simulink model "water_4hopper_VDF"  (Simulink 8.0)
settings: Solver=ode23  StartTime=0.0  StopTime=30  RelTol=1e-3
values from neighbouring files (symbols this model uses):
  alpha = 30    [SimParam_4VDF.m]
  Amp = leg_length    (= 0.0249)    [SimParam_4VDF.m]
  b_water = 0.5*C_d*S1*density    (= 0.405708731037)    [SimParam_4VDF.m]
  C_d = 0.703    [SimParam.m]    (also in SimParam_4VDF.m)
  density = 1000    [SimParam.m]    (also in SimParam_4VDF.m)
  frame_inertia = diag([Ix,Iy,Iz])    [SimParam.m]    (also in SimParam_4VDF.m)
  Fratio = 1/16    (= 0.0625)    [SimParam_4VDF.m]
  freq = 20    [SimParam.m]    (also in SimParam_4VDF.m = 60)
  g = 9.81    [SimParam.m]    (also in SimParam_4VDF.m)
  k_water = C_d*S1*density*g    (= 7.96000530294)    [SimParam_4VDF.m]
  leg_length = 0.06    [SimParam.m]    (also in SimParam_4VDF.m = 0.0249)
  Lx = frame_width/2*[-1 -1 1 1]'    [SimParam_4VDF.m]
  Lxmat = frame_width/2*[-1 0 0 0 ; 0 -1 0 0 ; 0 0 1 0 ; 0 0 0 1]    [SimParam_4VDF.m]
  Lz = frame_length/2*[-1 1 1 -1]'    [SimParam_4VDF.m]
  Lzmat = frame_length/2*[-1 0 0 0 ; 0 1 0 0 ; 0 0 1 0 ; 0 0 0 -1]    [SimParam_4VDF.m]
  mass = 0.1    [SimParam.m]    (also in SimParam_4VDF.m)
  mass_matrix = [mass 0 0; 0 Ix 0 ; 0 0 Iz]    [SimParam_4VDF.m]
  omega_0 = freq*ones(8,1)    [SimParam_4VDF.m]
  S1 = pi*r1^2    (= 0.00125663706144)    [SimParam.m]    (also in SimParam_4VDF.m = 0.00115422114093)
  S2 = pi*r2^2    (= 7.85398163397e-05)    [SimParam.m]    (also in SimParam_4VDF.m = 7.21388213081e-05)
  tau = 0.005    [SimParam_4VDF.m]
  wave = eps    [SimParam_4VDF.m]
  wavefreq = .5    (= 0.5)    [SimParam_4VDF.m]
undefined symbols (not defined in the file): amp, cw_FL_HL, cw_FR_FL, cw_FR_HR, cw_HR_HL, Filter_Coef, FL_HL_lag, FR_FL_lag, FR_HR_lag, HR_HL_lag, K_d, K_i, K_p, y_0
libraries: mblibv1 x34, dspstat3 x6, dspinverses x1
(part 1 of 2)
settings Model: Creator=Metti  LastModifiedBy=nitisht  SimulationMode=accelerator
settings SolverCC: ZeroCrossControl=DisableAll
settings DataIOCC: SignalLoggingSaveFormat=ModelDataLogs
settings DebuggingCC: FcnCallInpInsideContextMsg=EnableAllAsWarning
settings SimMechanicsCC: VisSampleTime=0.05  AutoFitVis=GROWTOFIT  LastVizWinPosition=[1 41 1600 759]  CamPosition=[-6.20117;3.01965;9.86212;]  CamTarget=[-0.265896;0.0450483;0.16365;]  CamUpVector=[0.0887544;0.966202;-0.242026;]  CamHeight=0.984746  VisBackgroundColor=[0.9;0.9;0.95;]  DefaultBodyColor=[1;0;0;]
settings ConfigurationSet: Description=SimMechanics 2G

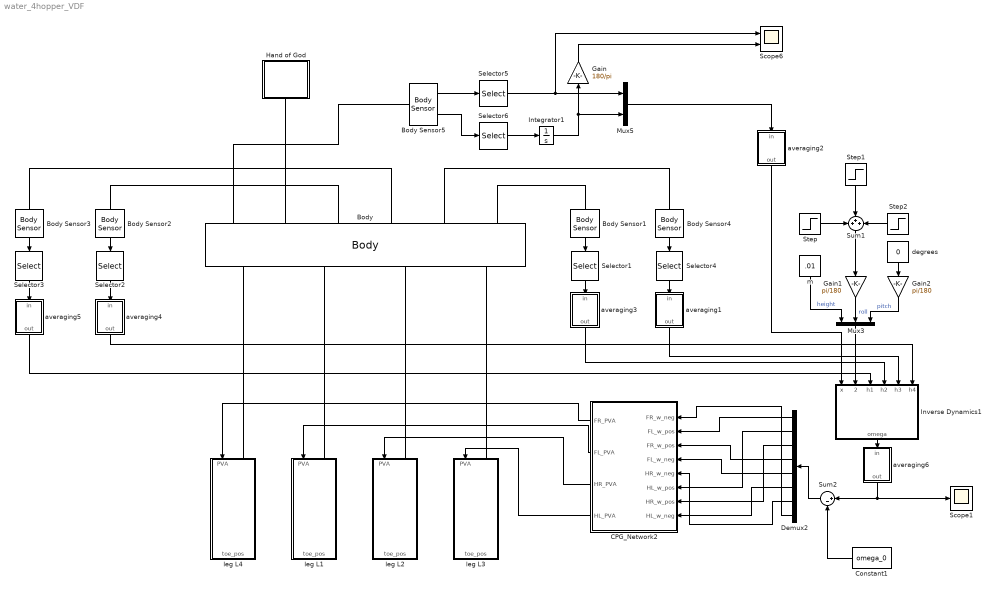
== system water_4hopper_VDF ==
  Body : mblibv1/Bodies/Body  LConnTagsString=CG|CS1|CS6|CS7|CS8|CS9  RConnTagsString=CS2|CS3|CS4|CS5  UpdateFromCAD=off  DialogClass=MechanicalBodyBlock  Mass=mass  MassUnits=kg  InertiaUnits=kg*m^2  Inertia=frame_inertia  Shape=Cylinder  ShapeDims=[1 1]  ShapeUnits=m  ShapeUse=false  Density=1  DensityUnits=kg/m^3  DensityUse=false  GraphicsMode=MACHINE_DEFAULT  BodyColorSelMode=MACHINE_DEFAULT  BodyColor=[1 0 0]  AttachedToCS=CG  CG=Left$CG$CG_pos$CS1$CS1$m$[0 0 0]$Euler X-Y-Z$deg$WORLD$true$none  WorkingFrames=Left$CS1$[0 0 0]$Adjoining$Adjoining$m$[0 0 0]$Euler X-Y-Z$deg$WORLD$true$none#Right$CS2$TR_FR$CS1$CS1$m$[0 0 0]$Euler X-Y-Z$deg$WORLD$true$none#Left$CS6$TR_FR$CS1$CS1$m$[0 0 0]$Euler X-Y-Z$deg$WORLD$true$none#Right$CS3$TR_FL$CS1$CS1$m$[0 0 0]$Euler X-Y-Z$deg$WORLD$true$none#Left$CS7$TR_FL$CS1$CS1$m$[0 0 0]$Euler X-Y-Z$deg$WORLD$true$none#Right$CS4$TR_HR$CS1$CS1$m$[0 0 0]$Euler X-Y-Z$deg$WORLD$true$none#Left$CS8$TR_HR$CS1$CS1$m$[0 0 0]$Euler X-Y-Z$deg$WORLD$true$none#Right$CS5$TR_HL$CS1$CS1$m$[0 0 0]$Euler X-Y-Z$deg$WORLD$true$none#Left$CS9$TR_HL$CS1$CS1$m$[0 0 0]$Euler X-Y-Z$deg$WORLD$true$none  CGPos=CG_pos  CGRot=[0 0 0]  CS0Pos=[]  CS0Rot=[]  CS1Pos=[0 0 0]  CS1Rot=[0 0 0]  CS2Pos=TR_FR  CS2Rot=[0 0 0]  CS3Pos=TR_FL  CS3Rot=[0 0 0]  CS4Pos=TR_HR  CS4Rot=[0 0 0]  CS5Pos=TR_HL  CS5Rot=[0 0 0]  CS6Pos=TR_FR  CS6Rot=[0 0 0]  CS7Pos=TR_FL  CS7Rot=[0 0 0]  CS8Pos=TR_HR  CS8Rot=[0 0 0]  CS9Pos=TR_HL  CS9Rot=[0 0 0]  CS10Pos=[]  CS10Rot=[]  CS11Pos=[]  CS11Rot=[]  CS12Pos=[]  CS12Rot=[]  CS13Pos=[]  CS13Rot=[]  CS14Pos=[]  CS14Rot=[]  CS15Pos=[]  CS15Rot=[]  CS16Pos=[]  CS16Rot=[]  CS17Pos=[]  CS17Rot=[]  CS18Pos=[]  CS18Rot=[]  CS19Pos=[]  CS19Rot=[]  CS20Pos=[]  CS20Rot=[]
  Body Sensor{1..4} (4 alike) : mblibv1/Sensors &  Actuators/Body Sensor  UpdateFromCAD=off  PhysicalDomain=Mechanical  PortType=blob  Muxed=on  Pose=off  Angle=on  AngleUnits=deg  ArcVelocity=off  ArcVelocityUnits=deg/s  ArcAcceleration=off  ArcAccelerationUnits=deg/s^2  CoordPosition=on  CoordPositionUnits=m  Velocity=off  VelocityUnits=m/s  Acceleration=off  AccelerationUnits=m/s^2  Quaternion=on  QuaternionDT=off  QuaternionDDT=off  QuaternionUnits=off  OutputVector=[1]  ActiveIO=on  Width=3  DialogClass=MechanicalSensorBlock  ReferenceFrame=Absolute (World)
  Body Sensor5 : mblibv1/Sensors &  Actuators/Body Sensor  UpdateFromCAD=off  PhysicalDomain=Mechanical  PortType=blob  Muxed=off  Pose=off  Angle=on  AngleUnits=deg  ArcVelocity=on  ArcVelocityUnits=rad/s  ArcAcceleration=off  ArcAccelerationUnits=deg/s^2  CoordPosition=on  CoordPositionUnits=m  Velocity=off  VelocityUnits=m/s  Acceleration=off  AccelerationUnits=m/s^2  Quaternion=on  QuaternionDT=off  QuaternionDDT=off  QuaternionUnits=off  OutputVector=[1]  ActiveIO=on  Width=6  DialogClass=MechanicalSensorBlock  ReferenceFrame=Absolute (World)
  CPG_Network2 : Subsystem
  Constant1 : Constant  Value=omega_0
  Demux2 : Demux  Outputs=8
  Gain : Gain  Gain=180/pi
  Gain1 : Gain  Gain=pi/180
  Gain2 : Gain  Gain=pi/180
  Hand of God : Subsystem
  Integrator1 : Integrator
  Inverse Dynamics1 : Subsystem
  Mux3 : Mux  Inputs=3
  Mux5 : Mux  Inputs=2
  Scope1 : Scope
      settings: TimeRange=30  YMin=5  YMax=105  SaveName=ball_position1
  Scope6 : Scope  NumInputPorts=2
      settings: TimeRange=30  YMin=-0.015~-17.5  YMax=0.065~15  SaveName=ball_position
  Selector{1..5} (5 alike) : Selector  InputPortWidth=3  IndexOptions=Index vector (dialog)  Indices=[2]  OutputSizes=1
  Selector6 : Selector  InputPortWidth=3  IndexOptions=Index vector (dialog)  Indices=[1 3]  OutputSizes=1
  Step : Step  Time=5  After=5  SampleTime=0
  Step1 : Step  Time=10  After=-10  SampleTime=0
  Step2 : Step  Time=15  After=5  SampleTime=0
  Sum1 : Sum  Inputs=+++
  Sum2 : Sum  Inputs=|+-
  averaging1 : Subsystem  mask{T_win=2*pi/freq*4, x_init=[y_0-leg_length, 0, 0]}
      mask prompts: T_win "window (s)"; x_init "Initial condition"
  averaging2 : Subsystem  mask{T_win=2*pi/freq*4, x_init=[y_0, 0, 0]}
      mask prompts: T_win "window (s)"; x_init "Initial condition"
  averaging3 : Subsystem  mask{T_win=2*pi/freq*4, x_init=[y_0-leg_length, 0, 0]}
      mask prompts: T_win "window (s)"; x_init "Initial condition"
  averaging4 : Subsystem  mask{T_win=2*pi/freq*4, x_init=[y_0-leg_length, 0, 0]}
      mask prompts: T_win "window (s)"; x_init "Initial condition"
  averaging5 : Subsystem  mask{T_win=2*pi/freq*4, x_init=[y_0-leg_length, 0, 0]}
      mask prompts: T_win "window (s)"; x_init "Initial condition"
  averaging6 : Subsystem  mask{T_win=2*pi/freq, x_init=omega_0}
      mask prompts: T_win "window (s)"; x_init "Initial condition"
  degrees : Constant  Value=0
  leg L1 : Subsystem  mask{seed=1}
      mask prompts: seed "random number seed"
  leg L2 : Subsystem  mask{seed=2}
      mask prompts: seed "random number seed"
  leg L3 : Subsystem  mask{seed=3}
      mask prompts: seed "random number seed"
  leg L4 : Subsystem  mask{seed=0}
      mask prompts: seed "random number seed"
  m : Constant  Value=.01
  wires:
  Body Sensor1/1 -> Selector1/1
  Body Sensor4/1 -> Selector4/1
  m/1 -> Mux3/1  "height"
  Mux3/1 -> Inverse Dynamics1/2(x_des)
  Selector5/1 -> Scope6/1, Mux5/1
  Integrator1/1 -> Mux5/2, Gain/1
  Body Sensor2/1 -> Selector2/1
  Body Sensor3/1 -> Selector3/1
  Body Sensor5/1 -> Selector5/1
  Body Sensor5/2 -> Selector6/1
  Selector6/1 -> Integrator1/1
  Constant1/1 -> Sum2/2
  Sum2/1 -> Demux2/1
  Demux2/1 -> CPG_Network2/2(FL_w_pos)
  Demux2/5 -> CPG_Network2/4(FL_w_neg)
  Demux2/2 -> CPG_Network2/6(HL_w_pos)
  Demux2/6 -> CPG_Network2/8(HL_w_neg)
  Demux2/3 -> CPG_Network2/7(HR_w_pos)
  Demux2/7 -> CPG_Network2/5(HR_w_neg)
  Demux2/4 -> CPG_Network2/3(FR_w_pos)
  Demux2/8 -> CPG_Network2/1(FR_w_neg)
  CPG_Network2/1(FR_PVA) -> leg L4/1(PVA)
  CPG_Network2/2(FL_PVA) -> leg L1/1(PVA)
  CPG_Network2/3(HR_PVA) -> leg L2/1(PVA)
  CPG_Network2/4(HL_PVA) -> leg L3/1(PVA)
  Gain/1 -> Scope6/2
  Gain1/1 -> Mux3/2  "roll"
  Gain2/1 -> Mux3/3  "pitch"
  Mux5/1 -> averaging2/1(in)
  averaging2/1(out) -> Inverse Dynamics1/1(x)
  Selector4/1 -> averaging1/1(in)
  Selector1/1 -> averaging3/1(in)
  Selector2/1 -> averaging4/1(in)
  Selector3/1 -> averaging5/1(in)
  averaging5/1(out) -> Inverse Dynamics1/3(h1)
  averaging4/1(out) -> Inverse Dynamics1/6(h4)
  averaging3/1(out) -> Inverse Dynamics1/4(h2)
  averaging1/1(out) -> Inverse Dynamics1/5(h3)
  Step/1 -> Sum1/1
  Step1/1 -> Sum1/2
  Step2/1 -> Sum1/3
  Inverse Dynamics1/1(omega) -> averaging6/1(in)
  averaging6/1(out) -> Sum2/1, Scope1/1
  degrees/1 -> Gain2/1
  Sum1/1 -> Gain1/1
  connections:
  Hand of God/RConn1 -- Body/LConn2
  Body/LConn6 -- Body Sensor1/LConn1
  Body/LConn5 -- Body Sensor4/LConn1
  Body/LConn1 -- Body Sensor5/LConn1
  leg L3/LConn1 -- Body/RConn4
  leg L2/LConn1 -- Body/RConn3
  leg L1/LConn1 -- Body/RConn2
  leg L4/LConn1 -- Body/RConn1
  Body/LConn3 -- Body Sensor2/LConn1
  Body/LConn4 -- Body Sensor3/LConn1

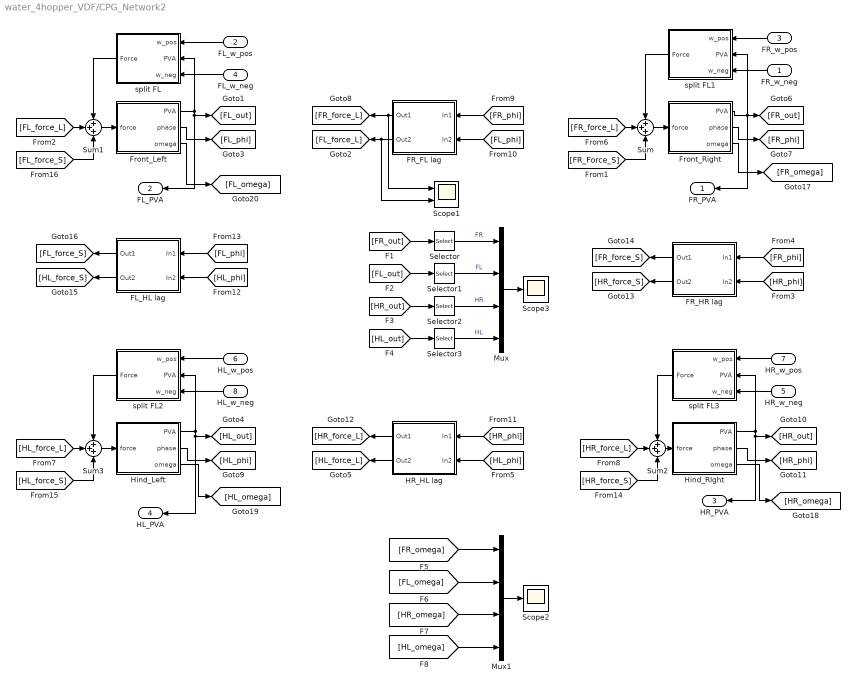
== system water_4hopper_VDF/CPG_Network2 ==
  FR_w_neg : Inport
  FL_w_pos : Inport  Port=2
  FR_w_pos : Inport  Port=3
  FL_w_neg : Inport  Port=4
  HR_w_neg : Inport  Port=5
  HL_w_pos : Inport  Port=6
  HR_w_pos : Inport  Port=7
  HL_w_neg : Inport  Port=8
  FL_HL lag : Subsystem  mask{d_phase=FL_HL_lag, coupling_weight=cw_FL_HL}
      mask prompts: d_phase "Phase Lag"; coupling_weight "Coupling Weight"
  FR_FL lag : Subsystem  mask{d_phase=FR_FL_lag, coupling_weight=cw_FR_FL}
      mask prompts: d_phase "Phase Lag"; coupling_weight "Coupling Weight"
  FR_HR lag : Subsystem  mask{d_phase=FR_HR_lag, coupling_weight=cw_FR_HR}
      mask prompts: d_phase "Phase Lag"; coupling_weight "Coupling Weight"
  Front_Left : Subsystem  mask{Amp=amp, Offset=0, init_phi=pi}
      mask prompts: Amp "Amplitude"; init_phi "Initial Phase"
  Front_Right : Subsystem  mask{Amp=amp, Offset=0, init_phi=0}
      mask prompts: Amp "Amplitude"; init_phi "Initial Phase"
  HR_HL lag : Subsystem  mask{d_phase=HR_HL_lag, coupling_weight=cw_HR_HL}
      mask prompts: d_phase "Phase Lag"; coupling_weight "Coupling Weight"
  Hind_Left : Subsystem  mask{Amp=amp, Offset=0, init_phi=0}
      mask prompts: Amp "Amplitude"; init_phi "Initial Phase"
  Hind_RIght : Subsystem  mask{Amp=amp, Offset=0, init_phi=pi}
      mask prompts: Amp "Amplitude"; init_phi "Initial Phase"
  Mux : Mux
  Mux1 : Mux
  Scope1 : Scope  NumInputPorts=2
      settings: ShowLegends=on  TimeRange=10  YMin=0~-5  YMax=2~5  SaveName=Output1
  Scope2 : Scope
      settings: ShowLegends=on  TimeRange=30  YMin=-20  YMax=130  SaveName=Output2
  Scope3 : Scope
      settings: ShowLegends=on  TimeRange=10  YMin=-0.025  YMax=0.025  SaveName=Output
  Selector{,1..3} (4 alike) : Selector  InputPortWidth=3  IndexOptions=Index vector (dialog)  Indices=[1]  OutputSizes=1
  Sum{,1..3} (4 alike) : Sum  Inputs=+++
  split FL : Subsystem
  split FL1 : Subsystem
  split FL2 : Subsystem
  split FL3 : Subsystem
  FR_PVA : Outport
  FL_PVA : Outport  Port=2
  HR_PVA : Outport  Port=3
  HL_PVA : Outport  Port=4
  wires:
  Mux/1 -> Scope3/1
  Front_Left/2(phase) -> [FL_phi]
  Front_Right/2(phase) -> [FR_phi]
  [FL_phi] -> FR_FL lag/2(In2)
  [FR_phi] -> FR_FL lag/1(In1)
  FR_FL lag/1(Out1) -> Scope1/1, [FR_force_L]
  FR_FL lag/2(Out2) -> Scope1/2, [FL_force_L]
  Front_Right/1(PVA) -> split FL1/2(PVA), FR_PVA/1, [FR_out]
  [FL_force_L] -> Sum1/2
  Sum1/1 -> Front_Left/1(force)
  Sum/1 -> Front_Right/1(force)
  [FR_force_L] -> Sum/2
  [FL_out] -> Selector1/1
  Selector1/1 -> Mux/2  "FL"
  Selector/1 -> Mux/1  "FR"
  [FR_out] -> Selector/1
  FR_w_pos/1 -> split FL1/1(w_pos)
  FR_w_neg/1 -> split FL1/3(w_neg)
  split FL1/1(Force) -> Sum/1
  FL_w_pos/1 -> split FL/1(w_pos)
  FL_w_neg/1 -> split FL/3(w_neg)
  Front_Left/1(PVA) -> FL_PVA/1, [FL_out], split FL/2(PVA)
  split FL/1(Force) -> Sum1/1
  Hind_Left/2(phase) -> [HL_phi]
  Hind_RIght/2(phase) -> [HR_phi]
  [HL_phi] -> HR_HL lag/2(In2)
  [HR_phi] -> HR_HL lag/1(In1)
  HR_HL lag/1(Out1) -> [HR_force_L]
  HR_HL lag/2(Out2) -> [HL_force_L]
  Hind_RIght/1(PVA) -> HR_PVA/1, [HR_out], split FL3/2(PVA)
  [HL_force_L] -> Sum3/2
  Sum3/1 -> Hind_Left/1(force)
  Sum2/1 -> Hind_RIght/1(force)
  [HR_force_L] -> Sum2/2
  HR_w_pos/1 -> split FL3/1(w_pos)
  HR_w_neg/1 -> split FL3/3(w_neg)
  split FL3/1(Force) -> Sum2/1
  HL_w_pos/1 -> split FL2/1(w_pos)
  HL_w_neg/1 -> split FL2/3(w_neg)
  Hind_Left/1(PVA) -> HL_PVA/1, [HL_out], split FL2/2(PVA)
  split FL2/1(Force) -> Sum3/1
  [HR_phi] -> FR_HR lag/2(In2)
  [FR_phi] -> FR_HR lag/1(In1)
  FR_HR lag/1(Out1) -> [FR_force_S]
  FR_HR lag/2(Out2) -> [HR_force_S]
  [HL_phi] -> FL_HL lag/2(In2)
  [FL_phi] -> FL_HL lag/1(In1)
  FL_HL lag/1(Out1) -> [FL_force_S]
  FL_HL lag/2(Out2) -> [HL_force_S]
  [HL_out] -> Selector3/1
  Selector3/1 -> Mux/4  "HL"
  Selector2/1 -> Mux/3  "HR"
  [HR_out] -> Selector2/1
  [FR_Force_S] -> Sum/3
  [HR_force_S] -> Sum2/3
  [HL_force_S] -> Sum3/3
  [FL_force_S] -> Sum1/3
  Front_Right/3(omega) -> [FR_omega]
  Hind_RIght/3(omega) -> [HR_omega]
  Hind_Left/3(omega) -> [HL_omega]
  Front_Left/3(omega) -> [FL_omega]
  Mux1/1 -> Scope2/1
  [FR_omega] -> Mux1/1
  [HL_omega] -> Mux1/4
  [HR_omega] -> Mux1/3
  [FL_omega] -> Mux1/2

== system water_4hopper_VDF/Hand of God ==
  Custom Joint : mblibv1/Joints/Custom Joint  LConnTagsString=__newl0|SA1  RConnTagsString=__newr0  UpdateFromCAD=off  NumSAPorts=1  CutJoint=off  MarkAsCut=off  Primitives=prismatic  PrimitiveProps=P1$World$[0 1 0]$Prismatic#R1$World$[1 0 0]$Revolute#R2$World$[0 0 1]$Revolute  DialogClass=JointBlock  R1Axis=[1 0 0]  R2Axis=[0 0 1]  R3Axis=[]  P1Axis=[0 1 0]  P2Axis=[]  P3Axis=[]  SAxis=[]
  Ground : mblibv1/Bodies/Ground  UpdateFromCAD=off  LeftPortType=env  RightPortType=workingframe  PhysicalDomain=Mechanical  DialogClass=GroundBlock  CoordPosition=[0 0 0]  CoordPositionUnits=m  StateVectorMgrId=3  MachineId=[4 0]  ShowEnvPort=on
  Joint Initial Condition : mblibv1/Sensors &  Actuators/Joint Initial Condition  UpdateFromCAD=off  LeftPortType=blob  RightPortType=blob  PhysicalDomain=mechanical  DialogClass=InitialConditionBlock  InitialConditions=P1$true$y_0$m$deg$0$m/s$deg/s#P2$false$0$m$deg$0$m/s$deg/s#P3$false$0$m$deg$0$m/s$deg/s#R1$true$0$m$deg$0$m/s$deg/s#R2$true$0$m$deg$0$m/s$deg/s#R3$false$10$m$deg$0$m/s$deg/s#S$false$0$m$deg$0$m/s$deg/s  P1PIC=y_0  P1VIC=0  P2PIC=0  P2VIC=0  P3PIC=0  P3VIC=0  R1PIC=0  R1VIC=0  R2PIC=0  R2VIC=0  R3PIC=0  R3VIC=0  SPIC=0  SVIC=0
  Joint Sensor : mblibv1/Sensors &  Actuators/Joint Sensor  UpdateFromCAD=off  PhysicalDomain=Mechanical  PortType=blob  Muxed=on  Pose=off  Angle=on  AngleUnits=deg  ArcVelocity=off  ArcVelocityUnits=deg/s  ArcAcceleration=off  ArcAccelerationUnits=deg/s^2  CoordPosition=on  CoordPositionUnits=m  Velocity=off  VelocityUnits=m/s  Acceleration=off  AccelerationUnits=m/s^2  Quaternion=on  QuaternionDT=off  QuaternionDDT=off  QuaternionUnits=off  OutputVector=[1]  ActiveIO=on  Width=1  DialogClass=MechanicalSensorBlock  Primitive=P1  Force=off  ForceUnits=N  Torque=off  TorqueUnits=N*m  ReferenceFrame=Absolute (World)  ReactionSensedSide=Base  ReactionReferenceFrame=Absolute (World)  ReactionForce=off  ReactionForceUnits=N  ReactionMoment=off  ReactionMomentUnits=N*m
  Joint Sensor1 : mblibv1/Sensors &  Actuators/Joint Sensor  UpdateFromCAD=off  PhysicalDomain=Mechanical  PortType=blob  Muxed=on  Pose=off  Angle=on  AngleUnits=deg  ArcVelocity=off  ArcVelocityUnits=deg/s  ArcAcceleration=off  ArcAccelerationUnits=deg/s^2  CoordPosition=off  CoordPositionUnits=m  Velocity=on  VelocityUnits=m/s  Acceleration=off  AccelerationUnits=m/s^2  Quaternion=on  QuaternionDT=off  QuaternionDDT=off  QuaternionUnits=off  OutputVector=[1]  ActiveIO=on  Width=1  DialogClass=MechanicalSensorBlock  Primitive=R1  Force=off  ForceUnits=N  Torque=off  TorqueUnits=N*m  ReferenceFrame=Absolute (World)  ReactionSensedSide=Base  ReactionReferenceFrame=Absolute (World)  ReactionForce=off  ReactionForceUnits=N  ReactionMoment=off  ReactionMomentUnits=N*m
  Joint Sensor2 : mblibv1/Sensors &  Actuators/Joint Sensor  UpdateFromCAD=off  PhysicalDomain=Mechanical  PortType=blob  Muxed=off  Pose=off  Angle=on  AngleUnits=deg  ArcVelocity=off  ArcVelocityUnits=deg/s  ArcAcceleration=off  ArcAccelerationUnits=deg/s^2  CoordPosition=on  CoordPositionUnits=m  Velocity=off  VelocityUnits=m/s  Acceleration=off  AccelerationUnits=m/s^2  Quaternion=on  QuaternionDT=off  QuaternionDDT=off  QuaternionUnits=off  OutputVector=[1]  ActiveIO=on  Width=1  DialogClass=MechanicalSensorBlock  Primitive=R2  Force=off  ForceUnits=N  Torque=off  TorqueUnits=N*m  ReferenceFrame=Absolute (World)  ReactionSensedSide=Base  ReactionReferenceFrame=Absolute (World)  ReactionForce=off  ReactionForceUnits=N  ReactionMoment=off  ReactionMomentUnits=N*m
  Machine Environment : mblibv1/Bodies/Machine Environment  PortType=env  PhysicalDomain=Mechanical  DialogTemplateClass=MECH.MachineEnvironment  SyncWhenCopied=off  Gravity=[0 -g 0]  GravityUnits=m/s^2  GravityAsSignal=off  Dimensionality=Auto-detect  AnalysisType=Forward dynamics  LinearAssemblyTolerance=1e-3  LinearAssemblyToleranceUnits=m  AngularAssemblyTolerance=1e-3  AngularAssemblyToleranceUnits=rad  ConstraintSolverType=Stabilizing  ConstraintRelTolerance=1e-4  ConstraintAbsTolerance=1e-4  UseRobustSingularityHandling=off  RedundancyAnalysisToleranceType=Automatically select tolerance  RedundancyAnalysisTolerance=1e-14  StatePerturbationType=Fixed  PerturbationSize=1e-5  VisualizeMachine=on  BodyVisualizationType=Use model default body geometries  BodyColorSelMode=Use model default  DefaultBodyColor=[1 0 0]
  Mechanical Branching Bar : mblibv1/Utilities/Mechanical Branching Bar  LConnTagsString=_newl0  RConnTagsString=__newr0|SA2|SA3|SA4  UpdateFromCAD=off  DialogClass=MechanicalBranchingBarBlock  NumSAPorts=4
  Scope : Scope  NumInputPorts=3
      settings: TimeRange=5  YMin=-0.01~-0.001~-6  YMax=0.02~0.0004~1  SaveName=mass_data
  Conn1 : PMIOPort  Port=1  Side=Right
  wires:
  Joint Sensor/1 -> Scope/1
  Joint Sensor1/1 -> Scope/2
  Joint Sensor2/1 -> Scope/3
  connections:
  Conn1/RConn1 -- Custom Joint/RConn1
  Joint Sensor1/LConn1 -- Mechanical Branching Bar/RConn3
  Ground/RConn1 -- Custom Joint/LConn1
  Machine Environment/RConn1 -- Ground/LConn1
  Joint Initial Condition/RConn1 -- Mechanical Branching Bar/RConn1
  Joint Sensor/LConn1 -- Mechanical Branching Bar/RConn2
  Custom Joint/LConn2 -- Mechanical Branching Bar/LConn1
  Joint Sensor2/LConn1 -- Mechanical Branching Bar/RConn4

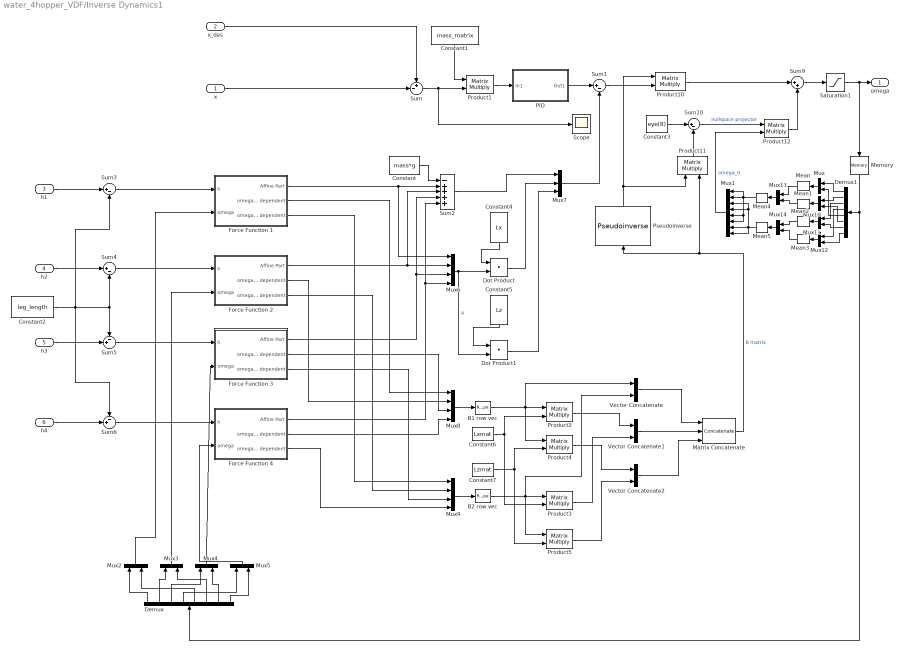
== system water_4hopper_VDF/Inverse Dynamics1 ==
  x : Inport
  x_des : Inport  Port=2
  h1 : Inport  Port=3
  h2 : Inport  Port=4
  h3 : Inport  Port=5
  h4 : Inport  Port=6
  B1 row vec : Reshape  OutputDimensionality=Row vector (2-D)  OutputDimensions=[1,2]
  B2 row vec : Reshape  OutputDimensionality=Row vector (2-D)  OutputDimensions=[1,2]
  Constant : Constant  Value=mass*g
  Constant1 : Constant  Value=mass_matrix
  Constant2 : Constant  Value=leg_length
  Constant3 : Constant  Value=eye(8)
  Constant4 : Constant  Value=Lx
  Constant5 : Constant  Value=Lz
  Constant6 : Constant  Value=Lxmat
  Constant7 : Constant  Value=Lzmat
  Demux : Demux  Outputs=8
  Demux1 : Demux  Outputs=8
  Dot Product : DotProduct  InputSameDT=on  OutDataTypeStr=Inherit: Inherit via internal rule
  Dot Product1 : DotProduct  InputSameDT=on  OutDataTypeStr=Inherit: Inherit via internal rule
  Force Function 1 : Subsystem
  Force Function 2 : Subsystem
  Force Function 3 : Subsystem
  Force Function 4 : Subsystem
  Matrix Concatenate : Concatenate  NumInputs=3  Mode=Multidimensional array
  Mean{,1..5} (6 alike) : dspstat3/Mean  run=off  reset_popup=None  InputProcessing=Columns as channels (frame based)  directionMode=Each column  dimension=1  treatSBRowAsCol=on  roiEnable=off  roiType=Rectangles  roiPortion=Entire ROI  roiOutput=Individual statistics for each ROI  roiFlag=off  outputDataTypeStr=Inherit: Same as accumulator  outputLastDataTypeStr=Inherit: Same as accumulator  outputMin=[]  outputMax=[]  roundingMode=Floor  overflowMode=off
  Memory : Memory  X0=omega_0
  Mux{,2..5,10..14} (10 alike) : Mux  Inputs=2
  Mux1 : Mux  Inputs=8
  Mux6 : Mux
  Mux7 : Mux  Inputs=3
  Mux8 : Mux
  Mux9 : Mux
  PID : Subsystem  mask{P=K_p, I=K_i, D=K_d, N=Filter_Coef}
      mask prompts: P "Proportional Gain"; I "Integral Gain"; D "Derivative Gain"; N "Filter Coefficient"
  Product{1..5,10..12} (8 alike) : Product  Multiplication=Matrix(*)  RndMeth=Zero
  Pseudoinverse : dspinverses/Pseudoinverse  wanterr=off
  Saturation1 : Saturate  UpperLimit=120  LowerLimit=10
  Scope : Scope
      settings: TimeRange=15  YMin=-0.01  YMax=0.09
  Sum : Sum  Inputs=+-|
  Sum{1,3..4,10} (4 alike) : Sum  Inputs=|+-
  Sum2 : Sum  Inputs=-++++
  Sum5 : Sum  Inputs=-+|
  Sum6 : Sum  Inputs=-+|
  Sum9 : Sum  Inputs=|++
  Vector Concatenate : Concatenate  ConcatenateDimension=2
  Vector Concatenate1 : Concatenate  ConcatenateDimension=2
  Vector Concatenate2 : Concatenate  ConcatenateDimension=2
  omega : Outport
  wires:
  Memory/1 -> Demux/1, Demux1/1
  PID/1(Out1) -> Sum1/1
  Sum/1 -> Scope/1, Product1/2
  x/1 -> Sum/2
  Pseudoinverse/1 -> Product11/1, Product10/1
  Sum1/1 -> Product10/2
  Product10/1 -> Sum9/1
  Product11/1 -> Sum10/2
  Constant3/1 -> Sum10/1
  Sum10/1 -> Product12/1  "nullspace projector"
  Product12/1 -> Sum9/2
  Mux1/1 -> Product12/2  "omega_0"
  Product1/1 -> PID/1(In1)
  Constant1/1 -> Product1/1
  Demux/1 -> Mux2/1
  Demux/5 -> Mux2/2
  Demux/2 -> Mux3/1
  Demux/6 -> Mux3/2
  Demux/3 -> Mux4/1
  Demux/7 -> Mux4/2
  Demux/4 -> Mux5/1
  Demux/8 -> Mux5/2
  Force Function 1/1(Affine Part) -> Mux6/1, Sum2/2
  Force Function 2/1(Affine Part) -> Sum2/3, Mux6/2
  Force Function 3/1(Affine Part) -> Mux6/3, Sum2/4
  Force Function 4/1(Affine Part) -> Mux6/4, Sum2/5
  Constant/1 -> Sum2/1
  Mux6/1 -> Dot Product/2, Dot Product1/2  "A"
  Constant4/1 -> Dot Product/1
  Constant5/1 -> Dot Product1/1
  Sum2/1 -> Mux7/1
  Dot Product/1 -> Mux7/2
  Dot Product1/1 -> Mux7/3
  Mux7/1 -> Sum1/2
  Force Function 1/2(omega1 dependent) -> Mux8/1
  Force Function 2/2(omega1 dependent) -> Mux8/2
  Force Function 3/2(omega1 dependent) -> Mux8/3
  Force Function 1/3(omega2 dependent) -> Mux9/1
  Force Function 2/3(omega2 dependent) -> Mux9/2
  Force Function 4/2(omega1 dependent) -> Mux8/4
  Force Function 3/3(omega2 dependent) -> Mux9/3
  Force Function 4/3(omega2 dependent) -> Mux9/4
  Mux8/1 -> B1 row vec/1
  Mux9/1 -> B2 row vec/1
  B1 row vec/1 -> Vector Concatenate/1, Product4/1, Product2/1
  B2 row vec/1 -> Vector Concatenate/2, Product5/1, Product3/1
  Constant6/1 -> Product3/2, Product2/2
  Constant7/1 -> Product4/2, Product5/2
  Product2/1 -> Vector Concatenate1/1
  Product3/1 -> Vector Concatenate1/2
  Product4/1 -> Vector Concatenate2/1
  Product5/1 -> Vector Concatenate2/2
  Vector Concatenate/1 -> Matrix Concatenate/1
  Vector Concatenate1/1 -> Matrix Concatenate/2
  Vector Concatenate2/1 -> Matrix Concatenate/3
  Matrix Concatenate/1 -> Product11/2, Pseudoinverse/1  "B matrix"
  Mux2/1 -> Force Function 1/2(omega)
  Mux3/1 -> Force Function 2/2(omega)
  Mux4/1 -> Force Function 3/2(omega)
  Mux5/1 -> Force Function 4/2(omega)
  h1/1 -> Sum3/1
  Sum3/1 -> Force Function 1/1(h)
  Sum4/1 -> Force Function 2/1(h)
  Sum5/1 -> Force Function 3/1(h)
  Sum6/1 -> Force Function 4/1(h)
  h2/1 -> Sum4/1
  h3/1 -> Sum5/2
  h4/1 -> Sum6/2
  Constant2/1 -> Sum3/2, Sum6/1, Sum5/1, Sum4/2
  x_des/1 -> Sum/1
  Sum9/1 -> Saturation1/1
  Saturation1/1 -> Memory/1, omega/1
  Demux1/1 -> Mux/1
  Mux/1 -> Mean/1
  Mux10/1 -> Mean1/1
  Mux11/1 -> Mean2/1
  Demux1/5 -> Mux/2
  Demux1/2 -> Mux10/1
  Demux1/6 -> Mux10/2
  Demux1/3 -> Mux11/1
  Demux1/7 -> Mux11/2
  Mux12/1 -> Mean3/1
  Demux1/4 -> Mux12/1
  Demux1/8 -> Mux12/2
  Mux13/1 -> Mean4/1
  Mean/1 -> Mux13/1
  Mean1/1 -> Mux13/2
  Mux14/1 -> Mean5/1
  Mean2/1 -> Mux14/1
  Mean3/1 -> Mux14/2
  Mean4/1 -> Mux1/6, Mux1/5, Mux1/2, Mux1/1
  Mean5/1 -> Mux1/8, Mux1/7, Mux1/4, Mux1/3

== system water_4hopper_VDF/averaging1 ==
  in : Inport
  Constant1 : Constant  Value=x_init
  Gain : Gain  Gain=1/T_win
  Integrator1 : Integrator
  Sum : Sum  Inputs=+-|
  Sum1 : Sum  Inputs=-+|
  Sum3 : Sum  Inputs=++|
  Transport Delay : TransportDelay  DelayTime=T_win
  out : Outport
  wires:
  in/1 -> Sum1/2
  Gain/1 -> Sum3/2
  Constant1/1 -> Sum3/1, Sum1/1
  Sum1/1 -> Integrator1/1
  Transport Delay/1 -> Sum/2
  Integrator1/1 -> Sum/1, Transport Delay/1
  Sum3/1 -> out/1
  Sum/1 -> Gain/1

== system water_4hopper_VDF/averaging2 ==
  in : Inport
  Constant1 : Constant  Value=x_init
  Gain : Gain  Gain=1/T_win
  Integrator1 : Integrator
  Sum : Sum  Inputs=+-|
  Sum1 : Sum  Inputs=-+|
  Sum3 : Sum  Inputs=++|
  Transport Delay : TransportDelay  DelayTime=T_win
  out : Outport
  wires:
  in/1 -> Sum1/2
  Gain/1 -> Sum3/2
  Constant1/1 -> Sum3/1, Sum1/1
  Sum1/1 -> Integrator1/1
  Transport Delay/1 -> Sum/2
  Integrator1/1 -> Sum/1, Transport Delay/1
  Sum3/1 -> out/1
  Sum/1 -> Gain/1

== system water_4hopper_VDF/averaging3 ==
  in : Inport
  Constant1 : Constant  Value=x_init
  Gain : Gain  Gain=1/T_win
  Integrator1 : Integrator
  Sum : Sum  Inputs=+-|
  Sum1 : Sum  Inputs=-+|
  Sum3 : Sum  Inputs=++|
  Transport Delay : TransportDelay  DelayTime=T_win
  out : Outport
  wires:
  in/1 -> Sum1/2
  Gain/1 -> Sum3/2
  Constant1/1 -> Sum3/1, Sum1/1
  Sum1/1 -> Integrator1/1
  Transport Delay/1 -> Sum/2
  Integrator1/1 -> Sum/1, Transport Delay/1
  Sum3/1 -> out/1
  Sum/1 -> Gain/1

== system water_4hopper_VDF/averaging4 ==
  in : Inport
  Constant1 : Constant  Value=x_init
  Gain : Gain  Gain=1/T_win
  Integrator1 : Integrator
  Sum : Sum  Inputs=+-|
  Sum1 : Sum  Inputs=-+|
  Sum3 : Sum  Inputs=++|
  Transport Delay : TransportDelay  DelayTime=T_win
  out : Outport
  wires:
  in/1 -> Sum1/2
  Gain/1 -> Sum3/2
  Constant1/1 -> Sum3/1, Sum1/1
  Sum1/1 -> Integrator1/1
  Transport Delay/1 -> Sum/2
  Integrator1/1 -> Sum/1, Transport Delay/1
  Sum3/1 -> out/1
  Sum/1 -> Gain/1

== system water_4hopper_VDF/averaging5 ==
  in : Inport
  Constant1 : Constant  Value=x_init
  Gain : Gain  Gain=1/T_win
  Integrator1 : Integrator
  Sum : Sum  Inputs=+-|
  Sum1 : Sum  Inputs=-+|
  Sum3 : Sum  Inputs=++|
  Transport Delay : TransportDelay  DelayTime=T_win
  out : Outport
  wires:
  in/1 -> Sum1/2
  Gain/1 -> Sum3/2
  Constant1/1 -> Sum3/1, Sum1/1
  Sum1/1 -> Integrator1/1
  Transport Delay/1 -> Sum/2
  Integrator1/1 -> Sum/1, Transport Delay/1
  Sum3/1 -> out/1
  Sum/1 -> Gain/1

== system water_4hopper_VDF/averaging6 ==
  in : Inport
  Constant1 : Constant  Value=x_init
  Gain : Gain  Gain=1/T_win
  Integrator1 : Integrator
  Sum : Sum  Inputs=+-|
  Sum1 : Sum  Inputs=-+|
  Sum3 : Sum  Inputs=++|
  Transport Delay : TransportDelay  DelayTime=T_win
  out : Outport
  wires:
  in/1 -> Sum1/2
  Gain/1 -> Sum3/2
  Constant1/1 -> Sum3/1, Sum1/1
  Sum1/1 -> Integrator1/1
  Transport Delay/1 -> Sum/2
  Integrator1/1 -> Sum/1, Transport Delay/1
  Sum3/1 -> out/1
  Sum/1 -> Gain/1

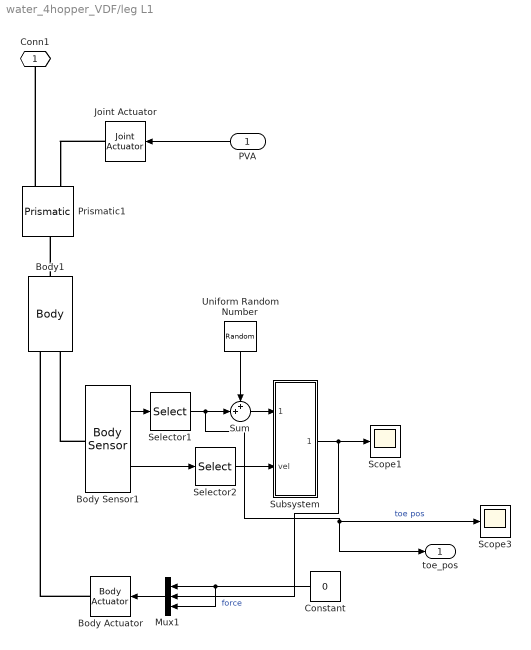
== system water_4hopper_VDF/leg L1 ==
  PVA : Inport
  Body Actuator : mblibv1/Sensors &  Actuators/Body Actuator  UpdateFromCAD=off  PhysicalDomain=Mechanical  PortType=blob  ActuationStyle=Force  AngleUnits=deg  ArcVelocityUnits=deg/s  ArcAccelerationUnits=deg/s^2  CoordPositionUnits=m  VelocityUnits=m/s  AccelerationUnits=m/s^2  ForceUnits=N  TorqueUnits=N*m  ActiveIO=on  Width=3  DialogClass=MechanicalActuatorBlock  ReferenceFrame=Absolute (World)  Angle=off  CoordPosition=on  Force=on  Torque=off
  Body Sensor1 : mblibv1/Sensors &  Actuators/Body Sensor  UpdateFromCAD=off  PhysicalDomain=Mechanical  PortType=blob  Muxed=off  Pose=off  Angle=on  AngleUnits=deg  ArcVelocity=off  ArcVelocityUnits=deg/s  ArcAcceleration=off  ArcAccelerationUnits=deg/s^2  CoordPosition=on  CoordPositionUnits=m  Velocity=on  VelocityUnits=m/s  Acceleration=off  AccelerationUnits=m/s^2  Quaternion=on  QuaternionDT=off  QuaternionDDT=off  QuaternionUnits=off  OutputVector=[1]  ActiveIO=on  Width=6  DialogClass=MechanicalSensorBlock  ReferenceFrame=Absolute (World)
  Body1 : mblibv1/Bodies/Body  LConnTagsString=CS1  RConnTagsString=CS2|CS3  UpdateFromCAD=off  DialogClass=MechanicalBodyBlock  Mass=0  MassUnits=kg  InertiaUnits=kg*m^2  Inertia=zeros(3)  Shape=Cylinder  ShapeDims=[1 1]  ShapeUnits=m  ShapeUse=false  Density=1  DensityUnits=kg/m^3  DensityUse=false  GraphicsMode=MACHINE_DEFAULT  BodyColorSelMode=MACHINE_DEFAULT  BodyColor=[1 0 0]  AttachedToCS=CG  CG=Left$CG$[0 -leg_length 0]$CS1$CS1$m$[0 0 0]$Euler X-Y-Z$deg$WORLD$false$none  WorkingFrames=Left$CS1$[0 0 0]$Adjoining$Adjoining$m$[0 0 0]$Euler X-Y-Z$deg$WORLD$true$none#Right$CS2$[0 -leg_length 0]$CS1$CS1$m$[0 0 0]$Euler X-Y-Z$deg$WORLD$true$none#Right$CS3$[0 -leg_length 0]$CS1$CS1$m$[0 0 0]$Euler X-Y-Z$deg$WORLD$true$none  CGPos=[0 -leg_length 0]  CGRot=[0 0 0]  CS0Pos=[]  CS0Rot=[]  CS1Pos=[0 0 0]  CS1Rot=[0 0 0]  CS2Pos=[0 -leg_length 0]  CS2Rot=[0 0 0]  CS3Pos=[0 -leg_length 0]  CS3Rot=[0 0 0]  CS4Pos=[]  CS4Rot=[]  CS5Pos=[]  CS5Rot=[]  CS6Pos=[]  CS6Rot=[]  CS7Pos=[]  CS7Rot=[]  CS8Pos=[]  CS8Rot=[]  CS9Pos=[]  CS9Rot=[]  CS10Pos=[]  CS10Rot=[]  CS11Pos=[]  CS11Rot=[]  CS12Pos=[]  CS12Rot=[]  CS13Pos=[]  CS13Rot=[]  CS14Pos=[]  CS14Rot=[]  CS15Pos=[]  CS15Rot=[]  CS16Pos=[]  CS16Rot=[]  CS17Pos=[]  CS17Rot=[]  CS18Pos=[]  CS18Rot=[]  CS19Pos=[]  CS19Rot=[]  CS20Pos=[]  CS20Rot=[]
  Constant : Constant  Value=0
  Joint Actuator : mblibv1/Sensors &  Actuators/Joint Actuator  UpdateFromCAD=off  PhysicalDomain=Mechanical  PortType=blob  ActuationStyle=Motion  AngleUnits=deg  ArcVelocityUnits=deg/s  ArcAccelerationUnits=deg/s^2  CoordPositionUnits=m  VelocityUnits=m/s  AccelerationUnits=m/s^2  ForceUnits=N  TorqueUnits=N*m  ActiveIO=on  Width=3  DialogClass=MechanicalActuatorBlock  Primitive=P1  ReferenceFrame=Absolute (World)
  Mux1 : Mux  Inputs=3
  Prismatic1 : mblibv1/Joints/Prismatic  LConnTagsString=__newl0|SA1  RConnTagsString=__newr0  UpdateFromCAD=off  NumSAPorts=1  CutJoint=off  MarkAsCut=off  Primitives=prismatic  PrimitiveProps=P1$World$[0 1 0]$prismatic  DialogClass=JointBlock  P1Axis=[0 1 0]
  Scope1 : Scope
      settings: SaveName=force_L
  Scope3 : Scope
      settings: SaveName=toe_position_L
  Selector1 : Selector  InputPortWidth=3  IndexOptions=Index vector (dialog)  Indices=[2]  OutputSizes=1
  Selector2 : Selector  InputPortWidth=3  IndexOptions=Index vector (dialog)  Indices=[2]  OutputSizes=1
  Subsystem : Subsystem
  Sum : Sum  Inputs=++|
  Uniform Random Number : UniformRandomNumber  Minimum=-wave  Maximum=wave  Seed=seed  SampleTime=1/wavefreq
  Conn1 : PMIOPort  Port=1  Side=Left
  toe_pos : Outport
  wires:
  Body Sensor1/2 -> Selector2/1
  Selector1/1 -> Sum/2, Scope3/1, toe_pos/1  "toe pos"
  Selector2/1 -> Subsystem/2(vel)
  Subsystem/1(force) -> Scope1/1, Mux1/2  "force"
  Mux1/1 -> Body Actuator/1
  Constant/1 -> Mux1/1, Mux1/3
  PVA/1 -> Joint Actuator/1
  Body Sensor1/1 -> Selector1/1
  Uniform Random Number/1 -> Sum/1
  Sum/1 -> Subsystem/1(pos)
  connections:
  Body1/LConn1 -- Prismatic1/RConn1
  Body Actuator/RConn1 -- Body1/RConn1
  Body Sensor1/LConn1 -- Body1/RConn2
  Prismatic1/LConn1 -- Conn1/RConn1
  Joint Actuator/RConn1 -- Prismatic1/LConn2

== system water_4hopper_VDF/leg L2 ==
  PVA : Inport
  Body Actuator : mblibv1/Sensors &  Actuators/Body Actuator  UpdateFromCAD=off  PhysicalDomain=Mechanical  PortType=blob  ActuationStyle=Force  AngleUnits=deg  ArcVelocityUnits=deg/s  ArcAccelerationUnits=deg/s^2  CoordPositionUnits=m  VelocityUnits=m/s  AccelerationUnits=m/s^2  ForceUnits=N  TorqueUnits=N*m  ActiveIO=on  Width=3  DialogClass=MechanicalActuatorBlock  ReferenceFrame=Absolute (World)  Angle=off  CoordPosition=on  Force=on  Torque=off
  Body Sensor1 : mblibv1/Sensors &  Actuators/Body Sensor  UpdateFromCAD=off  PhysicalDomain=Mechanical  PortType=blob  Muxed=off  Pose=off  Angle=on  AngleUnits=deg  ArcVelocity=off  ArcVelocityUnits=deg/s  ArcAcceleration=off  ArcAccelerationUnits=deg/s^2  CoordPosition=on  CoordPositionUnits=m  Velocity=on  VelocityUnits=m/s  Acceleration=off  AccelerationUnits=m/s^2  Quaternion=on  QuaternionDT=off  QuaternionDDT=off  QuaternionUnits=off  OutputVector=[1]  ActiveIO=on  Width=6  DialogClass=MechanicalSensorBlock  ReferenceFrame=Absolute (World)
  Body1 : mblibv1/Bodies/Body  LConnTagsString=CS1  RConnTagsString=CS2|CS3  UpdateFromCAD=off  DialogClass=MechanicalBodyBlock  Mass=0  MassUnits=kg  InertiaUnits=kg*m^2  Inertia=zeros(3)  Shape=Cylinder  ShapeDims=[1 1]  ShapeUnits=m  ShapeUse=false  Density=1  DensityUnits=kg/m^3  DensityUse=false  GraphicsMode=MACHINE_DEFAULT  BodyColorSelMode=MACHINE_DEFAULT  BodyColor=[1 0 0]  AttachedToCS=CG  CG=Left$CG$[0 -leg_length 0]$CS1$CS1$m$[0 0 0]$Euler X-Y-Z$deg$WORLD$false$none  WorkingFrames=Left$CS1$[0 0 0]$Adjoining$Adjoining$m$[0 0 0]$Euler X-Y-Z$deg$WORLD$true$none#Right$CS2$[0 -leg_length 0]$CS1$CS1$m$[0 0 0]$Euler X-Y-Z$deg$WORLD$true$none#Right$CS3$[0 -leg_length 0]$CS1$CS1$m$[0 0 0]$Euler X-Y-Z$deg$WORLD$true$none  CGPos=[0 -leg_length 0]  CGRot=[0 0 0]  CS0Pos=[]  CS0Rot=[]  CS1Pos=[0 0 0]  CS1Rot=[0 0 0]  CS2Pos=[0 -leg_length 0]  CS2Rot=[0 0 0]  CS3Pos=[0 -leg_length 0]  CS3Rot=[0 0 0]  CS4Pos=[]  CS4Rot=[]  CS5Pos=[]  CS5Rot=[]  CS6Pos=[]  CS6Rot=[]  CS7Pos=[]  CS7Rot=[]  CS8Pos=[]  CS8Rot=[]  CS9Pos=[]  CS9Rot=[]  CS10Pos=[]  CS10Rot=[]  CS11Pos=[]  CS11Rot=[]  CS12Pos=[]  CS12Rot=[]  CS13Pos=[]  CS13Rot=[]  CS14Pos=[]  CS14Rot=[]  CS15Pos=[]  CS15Rot=[]  CS16Pos=[]  CS16Rot=[]  CS17Pos=[]  CS17Rot=[]  CS18Pos=[]  CS18Rot=[]  CS19Pos=[]  CS19Rot=[]  CS20Pos=[]  CS20Rot=[]
  Constant : Constant  Value=0
  Joint Actuator : mblibv1/Sensors &  Actuators/Joint Actuator  UpdateFromCAD=off  PhysicalDomain=Mechanical  PortType=blob  ActuationStyle=Motion  AngleUnits=deg  ArcVelocityUnits=deg/s  ArcAccelerationUnits=deg/s^2  CoordPositionUnits=m  VelocityUnits=m/s  AccelerationUnits=m/s^2  ForceUnits=N  TorqueUnits=N*m  ActiveIO=on  Width=3  DialogClass=MechanicalActuatorBlock  Primitive=P1  ReferenceFrame=Absolute (World)
  Mux1 : Mux  Inputs=3
  Prismatic1 : mblibv1/Joints/Prismatic  LConnTagsString=__newl0|SA1  RConnTagsString=__newr0  UpdateFromCAD=off  NumSAPorts=1  CutJoint=off  MarkAsCut=off  Primitives=prismatic  PrimitiveProps=P1$World$[0 1 0]$prismatic  DialogClass=JointBlock  P1Axis=[0 1 0]
  Scope1 : Scope
      settings: SaveName=force_L
  Scope3 : Scope
      settings: SaveName=toe_position_L
  Selector1 : Selector  InputPortWidth=3  IndexOptions=Index vector (dialog)  Indices=[2]  OutputSizes=1
  Selector2 : Selector  InputPortWidth=3  IndexOptions=Index vector (dialog)  Indices=[2]  OutputSizes=1
  Subsystem : Subsystem
  Sum : Sum  Inputs=++|
  Uniform Random Number : UniformRandomNumber  Minimum=-wave  Maximum=wave  Seed=seed  SampleTime=1/wavefreq
  Conn1 : PMIOPort  Port=1  Side=Left
  toe_pos : Outport
  wires:
  Body Sensor1/2 -> Selector2/1
  Selector1/1 -> Sum/2, Scope3/1, toe_pos/1  "toe pos"
  Selector2/1 -> Subsystem/2(vel)
  Subsystem/1(force) -> Scope1/1, Mux1/2  "force"
  Mux1/1 -> Body Actuator/1
  Constant/1 -> Mux1/1, Mux1/3
  PVA/1 -> Joint Actuator/1
  Body Sensor1/1 -> Selector1/1
  Uniform Random Number/1 -> Sum/1
  Sum/1 -> Subsystem/1(pos)
  connections:
  Body1/LConn1 -- Prismatic1/RConn1
  Body Actuator/RConn1 -- Body1/RConn1
  Body Sensor1/LConn1 -- Body1/RConn2
  Prismatic1/LConn1 -- Conn1/RConn1
  Joint Actuator/RConn1 -- Prismatic1/LConn2

== system water_4hopper_VDF/leg L3 ==
  PVA : Inport
  Body Actuator : mblibv1/Sensors &  Actuators/Body Actuator  UpdateFromCAD=off  PhysicalDomain=Mechanical  PortType=blob  ActuationStyle=Force  AngleUnits=deg  ArcVelocityUnits=deg/s  ArcAccelerationUnits=deg/s^2  CoordPositionUnits=m  VelocityUnits=m/s  AccelerationUnits=m/s^2  ForceUnits=N  TorqueUnits=N*m  ActiveIO=on  Width=3  DialogClass=MechanicalActuatorBlock  ReferenceFrame=Absolute (World)  Angle=off  CoordPosition=on  Force=on  Torque=off
  Body Sensor1 : mblibv1/Sensors &  Actuators/Body Sensor  UpdateFromCAD=off  PhysicalDomain=Mechanical  PortType=blob  Muxed=off  Pose=off  Angle=on  AngleUnits=deg  ArcVelocity=off  ArcVelocityUnits=deg/s  ArcAcceleration=off  ArcAccelerationUnits=deg/s^2  CoordPosition=on  CoordPositionUnits=m  Velocity=on  VelocityUnits=m/s  Acceleration=off  AccelerationUnits=m/s^2  Quaternion=on  QuaternionDT=off  QuaternionDDT=off  QuaternionUnits=off  OutputVector=[1]  ActiveIO=on  Width=6  DialogClass=MechanicalSensorBlock  ReferenceFrame=Absolute (World)
  Body1 : mblibv1/Bodies/Body  LConnTagsString=CS1  RConnTagsString=CS2|CS3  UpdateFromCAD=off  DialogClass=MechanicalBodyBlock  Mass=0  MassUnits=kg  InertiaUnits=kg*m^2  Inertia=zeros(3)  Shape=Cylinder  ShapeDims=[1 1]  ShapeUnits=m  ShapeUse=false  Density=1  DensityUnits=kg/m^3  DensityUse=false  GraphicsMode=MACHINE_DEFAULT  BodyColorSelMode=MACHINE_DEFAULT  BodyColor=[1 0 0]  AttachedToCS=CG  CG=Left$CG$[0 -leg_length 0]$CS1$CS1$m$[0 0 0]$Euler X-Y-Z$deg$WORLD$false$none  WorkingFrames=Left$CS1$[0 0 0]$Adjoining$Adjoining$m$[0 0 0]$Euler X-Y-Z$deg$WORLD$true$none#Right$CS2$[0 -leg_length 0]$CS1$CS1$m$[0 0 0]$Euler X-Y-Z$deg$WORLD$true$none#Right$CS3$[0 -leg_length 0]$CS1$CS1$m$[0 0 0]$Euler X-Y-Z$deg$WORLD$true$none  CGPos=[0 -leg_length 0]  CGRot=[0 0 0]  CS0Pos=[]  CS0Rot=[]  CS1Pos=[0 0 0]  CS1Rot=[0 0 0]  CS2Pos=[0 -leg_length 0]  CS2Rot=[0 0 0]  CS3Pos=[0 -leg_length 0]  CS3Rot=[0 0 0]  CS4Pos=[]  CS4Rot=[]  CS5Pos=[]  CS5Rot=[]  CS6Pos=[]  CS6Rot=[]  CS7Pos=[]  CS7Rot=[]  CS8Pos=[]  CS8Rot=[]  CS9Pos=[]  CS9Rot=[]  CS10Pos=[]  CS10Rot=[]  CS11Pos=[]  CS11Rot=[]  CS12Pos=[]  CS12Rot=[]  CS13Pos=[]  CS13Rot=[]  CS14Pos=[]  CS14Rot=[]  CS15Pos=[]  CS15Rot=[]  CS16Pos=[]  CS16Rot=[]  CS17Pos=[]  CS17Rot=[]  CS18Pos=[]  CS18Rot=[]  CS19Pos=[]  CS19Rot=[]  CS20Pos=[]  CS20Rot=[]
  Constant : Constant  Value=0
  Joint Actuator : mblibv1/Sensors &  Actuators/Joint Actuator  UpdateFromCAD=off  PhysicalDomain=Mechanical  PortType=blob  ActuationStyle=Motion  AngleUnits=deg  ArcVelocityUnits=deg/s  ArcAccelerationUnits=deg/s^2  CoordPositionUnits=m  VelocityUnits=m/s  AccelerationUnits=m/s^2  ForceUnits=N  TorqueUnits=N*m  ActiveIO=on  Width=3  DialogClass=MechanicalActuatorBlock  Primitive=P1  ReferenceFrame=Absolute (World)
  Mux1 : Mux  Inputs=3
  Prismatic1 : mblibv1/Joints/Prismatic  LConnTagsString=__newl0|SA1  RConnTagsString=__newr0  UpdateFromCAD=off  NumSAPorts=1  CutJoint=off  MarkAsCut=off  Primitives=prismatic  PrimitiveProps=P1$World$[0 1 0]$prismatic  DialogClass=JointBlock  P1Axis=[0 1 0]
  Scope1 : Scope
      settings: SaveName=force_L
  Scope3 : Scope
      settings: SaveName=toe_position_L
  Selector1 : Selector  InputPortWidth=3  IndexOptions=Index vector (dialog)  Indices=[2]  OutputSizes=1
  Selector2 : Selector  InputPortWidth=3  IndexOptions=Index vector (dialog)  Indices=[2]  OutputSizes=1
  Subsystem : Subsystem
  Sum : Sum  Inputs=++|
  Uniform Random Number : UniformRandomNumber  Minimum=-wave  Maximum=wave  Seed=seed  SampleTime=1/wavefreq
  Conn1 : PMIOPort  Port=1  Side=Left
  toe_pos : Outport
  wires:
  Body Sensor1/2 -> Selector2/1
  Selector1/1 -> Sum/2, Scope3/1, toe_pos/1  "toe pos"
  Selector2/1 -> Subsystem/2(vel)
  Subsystem/1(force) -> Scope1/1, Mux1/2  "force"
  Mux1/1 -> Body Actuator/1
  Constant/1 -> Mux1/1, Mux1/3
  PVA/1 -> Joint Actuator/1
  Body Sensor1/1 -> Selector1/1
  Uniform Random Number/1 -> Sum/1
  Sum/1 -> Subsystem/1(pos)
  connections:
  Body1/LConn1 -- Prismatic1/RConn1
  Body Actuator/RConn1 -- Body1/RConn1
  Body Sensor1/LConn1 -- Body1/RConn2
  Prismatic1/LConn1 -- Conn1/RConn1
  Joint Actuator/RConn1 -- Prismatic1/LConn2

== system water_4hopper_VDF/leg L4 ==
  PVA : Inport
  Body Actuator : mblibv1/Sensors &  Actuators/Body Actuator  UpdateFromCAD=off  PhysicalDomain=Mechanical  PortType=blob  ActuationStyle=Force  AngleUnits=deg  ArcVelocityUnits=deg/s  ArcAccelerationUnits=deg/s^2  CoordPositionUnits=m  VelocityUnits=m/s  AccelerationUnits=m/s^2  ForceUnits=N  TorqueUnits=N*m  ActiveIO=on  Width=3  DialogClass=MechanicalActuatorBlock  ReferenceFrame=Absolute (World)  Angle=off  CoordPosition=on  Force=on  Torque=off
  Body Sensor1 : mblibv1/Sensors &  Actuators/Body Sensor  UpdateFromCAD=off  PhysicalDomain=Mechanical  PortType=blob  Muxed=off  Pose=off  Angle=on  AngleUnits=deg  ArcVelocity=off  ArcVelocityUnits=deg/s  ArcAcceleration=off  ArcAccelerationUnits=deg/s^2  CoordPosition=on  CoordPositionUnits=m  Velocity=on  VelocityUnits=m/s  Acceleration=off  AccelerationUnits=m/s^2  Quaternion=on  QuaternionDT=off  QuaternionDDT=off  QuaternionUnits=off  OutputVector=[1]  ActiveIO=on  Width=6  DialogClass=MechanicalSensorBlock  ReferenceFrame=Absolute (World)
  Body1 : mblibv1/Bodies/Body  LConnTagsString=CS1  RConnTagsString=CS2|CS3  UpdateFromCAD=off  DialogClass=MechanicalBodyBlock  Mass=0  MassUnits=kg  InertiaUnits=kg*m^2  Inertia=zeros(3)  Shape=Cylinder  ShapeDims=[1 1]  ShapeUnits=m  ShapeUse=false  Density=1  DensityUnits=kg/m^3  DensityUse=false  GraphicsMode=MACHINE_DEFAULT  BodyColorSelMode=MACHINE_DEFAULT  BodyColor=[1 0 0]  AttachedToCS=CG  CG=Left$CG$[0 -leg_length 0]$CS1$CS1$m$[0 0 0]$Euler X-Y-Z$deg$WORLD$false$none  WorkingFrames=Left$CS1$[0 0 0]$Adjoining$Adjoining$m$[0 0 0]$Euler X-Y-Z$deg$WORLD$true$none#Right$CS2$[0 -leg_length 0]$CS1$CS1$m$[0 0 0]$Euler X-Y-Z$deg$WORLD$true$none#Right$CS3$[0 -leg_length 0]$CS1$CS1$m$[0 0 0]$Euler X-Y-Z$deg$WORLD$true$none  CGPos=[0 -leg_length 0]  CGRot=[0 0 0]  CS0Pos=[]  CS0Rot=[]  CS1Pos=[0 0 0]  CS1Rot=[0 0 0]  CS2Pos=[0 -leg_length 0]  CS2Rot=[0 0 0]  CS3Pos=[0 -leg_length 0]  CS3Rot=[0 0 0]  CS4Pos=[]  CS4Rot=[]  CS5Pos=[]  CS5Rot=[]  CS6Pos=[]  CS6Rot=[]  CS7Pos=[]  CS7Rot=[]  CS8Pos=[]  CS8Rot=[]  CS9Pos=[]  CS9Rot=[]  CS10Pos=[]  CS10Rot=[]  CS11Pos=[]  CS11Rot=[]  CS12Pos=[]  CS12Rot=[]  CS13Pos=[]  CS13Rot=[]  CS14Pos=[]  CS14Rot=[]  CS15Pos=[]  CS15Rot=[]  CS16Pos=[]  CS16Rot=[]  CS17Pos=[]  CS17Rot=[]  CS18Pos=[]  CS18Rot=[]  CS19Pos=[]  CS19Rot=[]  CS20Pos=[]  CS20Rot=[]
  Constant : Constant  Value=0
  Joint Actuator : mblibv1/Sensors &  Actuators/Joint Actuator  UpdateFromCAD=off  PhysicalDomain=Mechanical  PortType=blob  ActuationStyle=Motion  AngleUnits=deg  ArcVelocityUnits=deg/s  ArcAccelerationUnits=deg/s^2  CoordPositionUnits=m  VelocityUnits=m/s  AccelerationUnits=m/s^2  ForceUnits=N  TorqueUnits=N*m  ActiveIO=on  Width=3  DialogClass=MechanicalActuatorBlock  Primitive=P1  ReferenceFrame=Absolute (World)
  Mux1 : Mux  Inputs=3
  Prismatic1 : mblibv1/Joints/Prismatic  LConnTagsString=__newl0|SA1  RConnTagsString=__newr0  UpdateFromCAD=off  NumSAPorts=1  CutJoint=off  MarkAsCut=off  Primitives=prismatic  PrimitiveProps=P1$World$[0 1 0]$prismatic  DialogClass=JointBlock  P1Axis=[0 1 0]
  Scope1 : Scope
      settings: SaveName=force_L
  Scope3 : Scope
      settings: SaveName=toe_position_L
  Selector1 : Selector  InputPortWidth=3  IndexOptions=Index vector (dialog)  Indices=[2]  OutputSizes=1
  Selector2 : Selector  InputPortWidth=3  IndexOptions=Index vector (dialog)  Indices=[2]  OutputSizes=1
  Subsystem : Subsystem
  Sum : Sum  Inputs=++|
  Uniform Random Number : UniformRandomNumber  Minimum=-wave  Maximum=wave  Seed=seed  SampleTime=1/wavefreq
  Conn1 : PMIOPort  Port=1  Side=Left
  toe_pos : Outport
  wires:
  Body Sensor1/2 -> Selector2/1
  Selector1/1 -> Sum/2, Scope3/1, toe_pos/1  "toe pos"
  Selector2/1 -> Subsystem/2(vel)
  Subsystem/1(force) -> Scope1/1, Mux1/2  "force"
  Mux1/1 -> Body Actuator/1
  Constant/1 -> Mux1/1, Mux1/3
  PVA/1 -> Joint Actuator/1
  Body Sensor1/1 -> Selector1/1
  Uniform Random Number/1 -> Sum/1
  Sum/1 -> Subsystem/1(pos)
  connections:
  Body1/LConn1 -- Prismatic1/RConn1
  Body Actuator/RConn1 -- Body1/RConn1
  Body Sensor1/LConn1 -- Body1/RConn2
  Prismatic1/LConn1 -- Conn1/RConn1
  Joint Actuator/RConn1 -- Prismatic1/LConn2

== system water_4hopper_VDF/CPG_Network2/FL_HL lag ==
  In1 : Inport
  In2 : Inport  Port=2
  Constant : Constant  Value=d_phase
  Gain : Gain  Gain=-1
  Sum : Sum  Inputs=--+
  sin : Fcn  Expr=coupling_weight*sin(u(1))
  Out1 : Outport
  Out2 : Outport  Port=2
  wires:
  Sum/1 -> sin/1
  sin/1 -> Gain/1, Out1/1
  Constant/1 -> Sum/2
  In1/1 -> Sum/1
  In2/1 -> Sum/3
  Gain/1 -> Out2/1

== system water_4hopper_VDF/CPG_Network2/FR_FL lag ==
  In1 : Inport
  In2 : Inport  Port=2
  Constant : Constant  Value=d_phase
  Gain : Gain  Gain=-1
  Sum : Sum  Inputs=--+
  sin : Fcn  Expr=coupling_weight*sin(u(1))
  Out1 : Outport
  Out2 : Outport  Port=2
  wires:
  Sum/1 -> sin/1
  sin/1 -> Gain/1, Out1/1
  Constant/1 -> Sum/2
  In1/1 -> Sum/1
  In2/1 -> Sum/3
  Gain/1 -> Out2/1

== system water_4hopper_VDF/CPG_Network2/FR_HR lag ==
  In1 : Inport
  In2 : Inport  Port=2
  Constant : Constant  Value=d_phase
  Gain : Gain  Gain=-1
  Sum : Sum  Inputs=--+
  sin : Fcn  Expr=coupling_weight*sin(u(1))
  Out1 : Outport
  Out2 : Outport  Port=2
  wires:
  Gain/1 -> Out2/1
  In2/1 -> Sum/3
  In1/1 -> Sum/1
  Constant/1 -> Sum/2
  sin/1 -> Out1/1, Gain/1
  Sum/1 -> sin/1

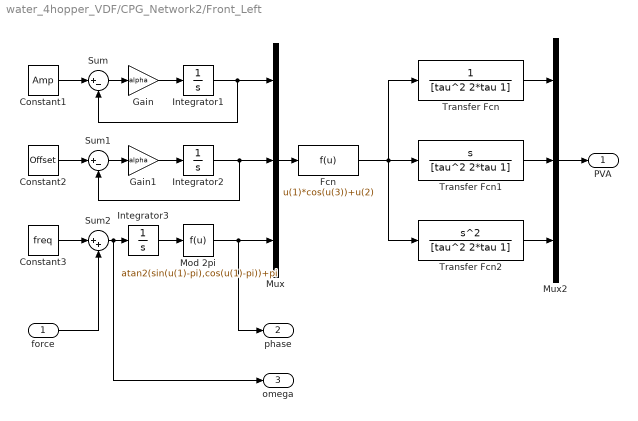
== system water_4hopper_VDF/CPG_Network2/Front_Left ==
  force : Inport
  Constant1 : Constant  Value=Amp
  Constant2 : Constant  Value=Offset
  Constant3 : Constant  Value=freq
  Fcn : Fcn  Expr=u(1)*cos(u(3))+u(2)
  Gain : Gain  Gain=alpha
  Gain1 : Gain  Gain=alpha
  Integrator1 : Integrator
  Integrator2 : Integrator
  Integrator3 : Integrator  InitialCondition=init_phi + 0.01*rand
  Mod 2pi : Fcn  Expr=atan2(sin(u(1)-pi),cos(u(1)-pi))+pi
  Mux : Mux  Inputs=3
  Mux2 : Mux  Inputs=3
  Sum : Sum  Inputs=|+-
  Sum1 : Sum  Inputs=|+-
  Sum2 : Sum  Inputs=|++
  Transfer Fcn : TransferFcn  Denominator=[tau^2 2*tau 1]
  Transfer Fcn1 : TransferFcn  Numerator=[1 0]  Denominator=[tau^2 2*tau 1]
  Transfer Fcn2 : TransferFcn  Numerator=[1 0 0]  Denominator=[tau^2 2*tau 1]
  PVA : Outport
  phase : Outport  Port=2
  omega : Outport  Port=3
  wires:
  Sum/1 -> Gain/1
  Integrator1/1 -> Sum/2, Mux/1
  Constant1/1 -> Sum/1
  Gain/1 -> Integrator1/1
  Sum1/1 -> Gain1/1
  Integrator2/1 -> Sum1/2, Mux/2
  Constant2/1 -> Sum1/1
  Gain1/1 -> Integrator2/1
  Mux/1 -> Fcn/1
  Mod 2pi/1 -> phase/1, Mux/3
  Integrator3/1 -> Mod 2pi/1
  Constant3/1 -> Sum2/1
  Sum2/1 -> omega/1, Integrator3/1
  force/1 -> Sum2/2
  Transfer Fcn2/1 -> Mux2/3
  Transfer Fcn/1 -> Mux2/1
  Transfer Fcn1/1 -> Mux2/2
  Fcn/1 -> Transfer Fcn2/1, Transfer Fcn/1, Transfer Fcn1/1
  Mux2/1 -> PVA/1

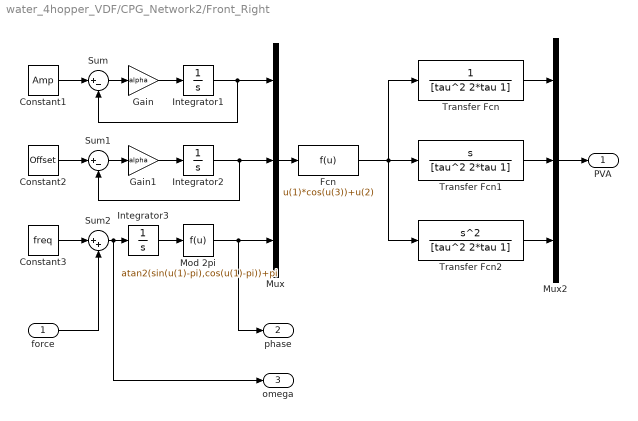
== system water_4hopper_VDF/CPG_Network2/Front_Right ==
  force : Inport
  Constant1 : Constant  Value=Amp
  Constant2 : Constant  Value=Offset
  Constant3 : Constant  Value=freq
  Fcn : Fcn  Expr=u(1)*cos(u(3))+u(2)
  Gain : Gain  Gain=alpha
  Gain1 : Gain  Gain=alpha
  Integrator1 : Integrator
  Integrator2 : Integrator
  Integrator3 : Integrator  InitialCondition=init_phi + 0.01*rand
  Mod 2pi : Fcn  Expr=atan2(sin(u(1)-pi),cos(u(1)-pi))+pi
  Mux : Mux  Inputs=3
  Mux2 : Mux  Inputs=3
  Sum : Sum  Inputs=|+-
  Sum1 : Sum  Inputs=|+-
  Sum2 : Sum  Inputs=|++
  Transfer Fcn : TransferFcn  Denominator=[tau^2 2*tau 1]
  Transfer Fcn1 : TransferFcn  Numerator=[1 0]  Denominator=[tau^2 2*tau 1]
  Transfer Fcn2 : TransferFcn  Numerator=[1 0 0]  Denominator=[tau^2 2*tau 1]
  PVA : Outport
  phase : Outport  Port=2
  omega : Outport  Port=3
  wires:
  Sum/1 -> Gain/1
  Integrator1/1 -> Sum/2, Mux/1
  Constant1/1 -> Sum/1
  Gain/1 -> Integrator1/1
  Sum1/1 -> Gain1/1
  Integrator2/1 -> Sum1/2, Mux/2
  Constant2/1 -> Sum1/1
  Gain1/1 -> Integrator2/1
  Mux/1 -> Fcn/1
  Mod 2pi/1 -> phase/1, Mux/3
  Integrator3/1 -> Mod 2pi/1
  Constant3/1 -> Sum2/1
  Sum2/1 -> omega/1, Integrator3/1
  force/1 -> Sum2/2
  Transfer Fcn2/1 -> Mux2/3
  Transfer Fcn/1 -> Mux2/1
  Transfer Fcn1/1 -> Mux2/2
  Fcn/1 -> Transfer Fcn2/1, Transfer Fcn/1, Transfer Fcn1/1
  Mux2/1 -> PVA/1

== system water_4hopper_VDF/CPG_Network2/HR_HL lag ==
  In1 : Inport
  In2 : Inport  Port=2
  Constant : Constant  Value=d_phase
  Gain : Gain  Gain=-1
  Sum : Sum  Inputs=--+
  sin : Fcn  Expr=coupling_weight*sin(u(1))
  Out1 : Outport
  Out2 : Outport  Port=2
  wires:
  Gain/1 -> Out2/1
  In2/1 -> Sum/3
  In1/1 -> Sum/1
  Constant/1 -> Sum/2
  sin/1 -> Out1/1, Gain/1
  Sum/1 -> sin/1
